simulink model "Full_Integration_Redundant"  (R2022b)
settings: Solver=ode15s  StartTime=0.0  StopTime=30  MaxStep=0.01  RelTol=1e-3
undefined symbols (not defined in the file): Bm1, Bm2, Br, Bsc, Btr, Continuous, G, Im1, Im2, Isw, Jtr, Ke, Ke2, Kl, kp, kr, ks, Ksc, Ksr, Kt, Kt2, ktr, Kv1, Kv2, L1, L2, lf, lr, Mr, N, n, n1, R1, R2, rp, Tfrc, Time, to, Vx, waypoints, z
libraries: simulink_extras x13, ctrlSharedLib x2, simulink x2, robotalgslib x1, slpidlib x1
settings Model: Creator=Timothy  LastModifiedBy=Timothy
settings DebuggingCC: SignalInfNanChecking=error

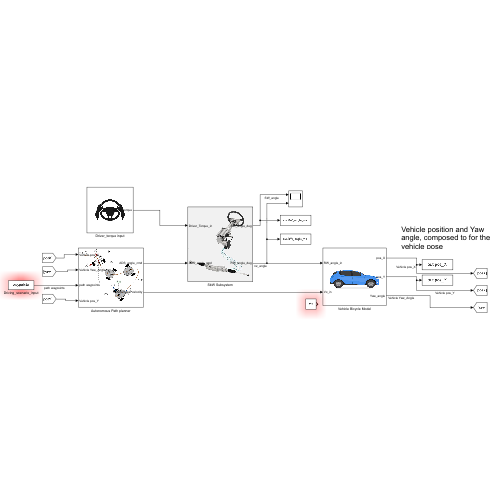
[thumbnail: Simulink's stored preview of the top-level diagram]
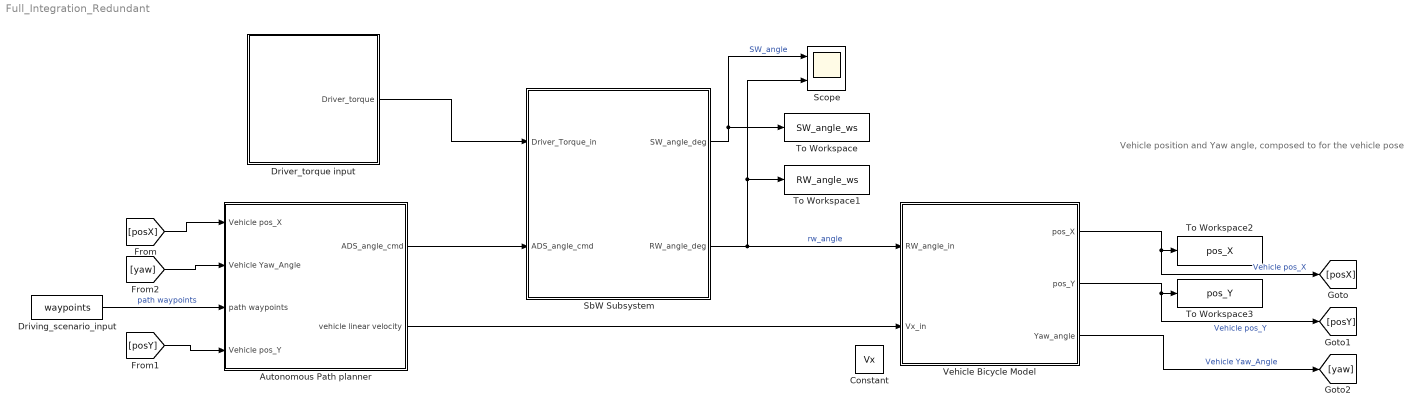
== system Full_Integration_Redundant ==
  note: Vehicle position and Yaw angle, composed to for the vehicle pose
  Autonomous Path planner : Subsystem
      mask Display: image('$imagefile'); % Use "Edit Image" on toolstrip to change.
  Constant : Constant  Value=Vx
  Driver_torque input : Subsystem
      mask Display: image('$imagefile'); % Use "Edit Image" on toolstrip to change.
  Driving_scenario_input : Constant  Value=waypoints
  SbW Subsystem : Subsystem
      mask Display: image('$imagefile'); % Use "Edit Image" on toolstrip to change.
  Scope : Scope  NumInputPorts=2
  To Workspace : ToWorkspace  VariableName=SW_angle_ws  SaveFormat=Timeseries  SampleTime=-1
  To Workspace1 : ToWorkspace  VariableName=RW_angle_ws  SaveFormat=Timeseries  SampleTime=-1
  To Workspace2 : ToWorkspace  VariableName=pos_X  SaveFormat=Timeseries  SampleTime=-1
  To Workspace3 : ToWorkspace  VariableName=pos_Y  SaveFormat=Timeseries  SampleTime=-1
  Vehicle Bicycle Model : Subsystem
      mask Display: image('$imagefile'); % Use "Edit Image" on toolstrip to change.
  wires:
  SbW Subsystem/1(SW_angle_deg) -> Scope/1, To Workspace/1  "SW_angle"
  Driving_scenario_input/1 -> Autonomous Path planner/3(path waypoints)  "path waypoints"
  Vehicle Bicycle Model/2(pos_Y) -> To Workspace3/1, [posY]  "Vehicle pos_Y"
  Autonomous Path planner/1(ADS_angle_cmd) -> SbW Subsystem/2(ADS_angle_cmd)
  Vehicle Bicycle Model/3(Yaw_angle) -> [yaw]  "Vehicle Yaw_Angle"
  SbW Subsystem/2(RW_angle_deg) -> Scope/2, To Workspace1/1, Vehicle Bicycle Model/1(RW_angle_in)  "rw_angle"
  Vehicle Bicycle Model/1(pos_X) -> [posX], To Workspace2/1  "Vehicle pos_X"
  [posX] -> Autonomous Path planner/1(Vehicle pos_X)
  [posY] -> Autonomous Path planner/4(Vehicle pos_Y)
  [yaw] -> Autonomous Path planner/2(Vehicle Yaw_Angle)
  Autonomous Path planner/2(vehicle linear velocity) -> Vehicle Bicycle Model/2(Vx_in)
  Driver_torque input/1(Driver_torque) -> SbW Subsystem/1(Driver_Torque_in)

== system Full_Integration_Redundant/Autonomous Path planner ==
  Vehicle pos_X : Inport
  Vehicle Yaw_Angle : Inport  Port=2
  path waypoints : Inport  Port=3
  Vehicle pos_Y : Inport  Port=4
  Angular converter : MATLAB Function  TreatAsAtomicUnit=on
  Mux : Mux  Inputs=3
  Pure Pursuit : robotalgslib/Pure Pursuit  DesiredLinearVelocity=1.7  MaxAngularVelocity=50  LookaheadDistance=1.0  TargetDirPort=off  SimulateUsing=Code generation
      settings: LibrarySourceBlock=robotmobilelib/Pure Pursuit
  Radians to Degrees : simulink_extras/Transformations/Radians to Degrees
  Scope3 : Scope
  ADS_angle_cmd : Outport
  vehicle linear velocity : Outport  Port=2
  wires:
  Vehicle pos_Y/1 -> Mux/2
  Pure Pursuit/1 -> vehicle linear velocity/1, Scope3/1, Angular converter/2(v)  "vehicle linear velocity"
  Vehicle Yaw_Angle/1 -> Mux/3
  Pure Pursuit/2 -> Angular converter/1(omega)
  Mux/1 -> Pure Pursuit/1  "vehicle_pose"
  Angular converter/1(delta) -> Radians to Degrees/1
  Radians to Degrees/1 -> ADS_angle_cmd/1  "ADS_angle_cmd"
  path waypoints/1 -> Pure Pursuit/2
  Vehicle pos_X/1 -> Mux/1

== system Full_Integration_Redundant/Driver_torque input ==
  note: The Driver torque configuration Can be entered here
  Add : Sum  Inputs=+-+-
  Step : Step  Time=0  SampleTime=0
  Step1 : Step  Time=0  After=0  SampleTime=0
  Step2 : Step  Time=0  After=0  SampleTime=0
  Step3 : Step  Time=0  After=0  SampleTime=0
  Driver_torque : Outport
  wires:
  Step/1 -> Add/1
  Add/1 -> Driver_torque/1  "Driver_torque"
  Step1/1 -> Add/2
  Step2/1 -> Add/3
  Step3/1 -> Add/4

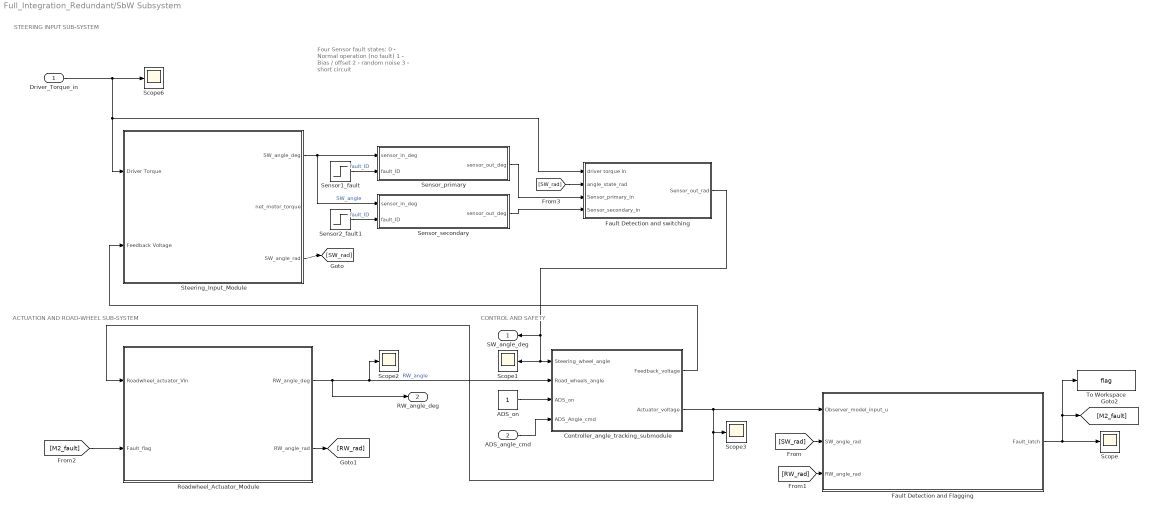
== system Full_Integration_Redundant/SbW Subsystem ==
  note: CONTROL AND SAFETY
  note: Four Sensor fault states:
      | 0 - Normal operation (no fault)
      | 1 - Bias / offset
      | 2 - random noise
      | 3 - short circuit
  note: ACTUATION AND ROAD-WHEEL SUB-SYSTEM
  note: STEERING INPUT SUB-SYSTEM
  Driver_Torque_in : Inport
  ADS_angle_cmd : Inport  Port=2
  ADS_on : Constant
  Controller_angle_tracking_submodule : Subsystem
  Fault Detection and Flagging : Subsystem
  Fault Detection and switching : Subsystem
  Roadwheel_Actuator_Module : Subsystem
  Scope{,1..3,6} (5 alike) : Scope
  Sensor1_fault : Step  SampleTime=0
  Sensor2_fault1 : Step  SampleTime=0
  Sensor_primary : Subsystem
  Sensor_secondary : Subsystem
  Steering_Input_Module : Subsystem
  To Workspace : ToWorkspace  VariableName=flag  SaveFormat=Timeseries  SampleTime=-1
  SW_angle_deg : Outport
  RW_angle_deg : Outport  Port=2
  wires:
  Roadwheel_Actuator_Module/1(RW_angle_deg) -> Controller_angle_tracking_submodule/2(Road_wheels_angle), Scope2/1, RW_angle_deg/1  "RW_angle"
  Controller_angle_tracking_submodule/2(Actuator_voltage) -> Fault Detection and Flagging/1(Observer_model_input_u), Roadwheel_Actuator_Module/1(Roadwheel_actuator_Vin), Scope3/1
  Controller_angle_tracking_submodule/1(Feedback_voltage) -> Steering_Input_Module/2(Feedback Voltage)
  Driver_Torque_in/1 -> Fault Detection and switching/1(driver torque in), Steering_Input_Module/1(Driver Torque), Scope6/1
  Steering_Input_Module/3(SW_angle_rad) -> [SW_rad]
  Roadwheel_Actuator_Module/2(RW_angle_rad) -> [RW_rad]
  Fault Detection and Flagging/1(Fault_latch) -> Scope/1, To Workspace/1, [M2_fault]
  ADS_on/1 -> Controller_angle_tracking_submodule/3(ADS_on)
  ADS_angle_cmd/1 -> Controller_angle_tracking_submodule/4(ADS_Angle_cmd)
  [SW_rad] -> Fault Detection and Flagging/2(SW_angle_rad)
  [RW_rad] -> Fault Detection and Flagging/3(RW_angle_rad)
  [M2_fault] -> Roadwheel_Actuator_Module/2(Fault_flag)
  Sensor1_fault/1 -> Sensor_primary/2(fault_ID)  "fault_ID"
  Sensor2_fault1/1 -> Sensor_secondary/2(fault_ID)  "fault_ID"
  [SW_rad] -> Fault Detection and switching/2(angle_state_rad)
  Sensor_primary/1(sensor_out_deg) -> Fault Detection and switching/3(Sensor_primary_in)
  Sensor_secondary/1(sensor_out_deg) -> Fault Detection and switching/4(Sensor_secondary_in)
  Steering_Input_Module/1(SW_angle_deg) -> Sensor_secondary/1(sensor_in_deg), Sensor_primary/1(sensor_in_deg)  "SW_angle"
  Fault Detection and switching/1(Sensor_out_rad) -> SW_angle_deg/1, Scope1/1, Controller_angle_tracking_submodule/1(Steering_wheel_angle)

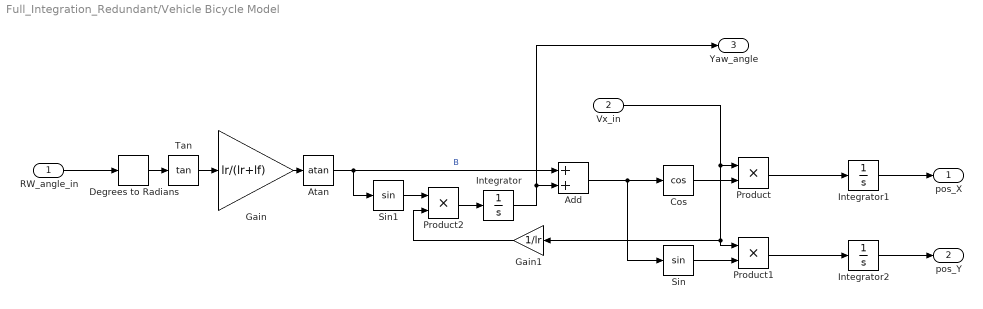
== system Full_Integration_Redundant/Vehicle Bicycle Model ==
  RW_angle_in : Inport
  Vx_in : Inport  Port=2
  Add : Sum
  Atan : Trigonometry  Operator=atan
  Cos : Trigonometry  Operator=cos
  Degrees to Radians : simulink_extras/Transformations/Degrees to Radians
  Gain : Gain  Gain=lr/(lr+lf)
  Gain1 : Gain  Gain=1/lr
  Integrator : Integrator
  Integrator1 : Integrator
  Integrator2 : Integrator
  Product : Product
  Product1 : Product
  Product2 : Product
  Sin : Trigonometry
  Sin1 : Trigonometry
  Tan : Trigonometry  Operator=tan
  pos_X : Outport
  pos_Y : Outport  Port=2
  Yaw_angle : Outport  Port=3
  wires:
  Degrees to Radians/1 -> Tan/1
  Product2/1 -> Integrator/1
  Cos/1 -> Product/2
  Add/1 -> Sin/1, Cos/1
  Atan/1 -> Add/1, Sin1/1  "B"
  Vx_in/1 -> Product1/1, Gain1/1, Product/1
  Integrator1/1 -> pos_X/1
  Gain1/1 -> Product2/2
  Integrator/1 -> Yaw_angle/1, Add/2
  Integrator2/1 -> pos_Y/1
  Gain/1 -> Atan/1
  Product/1 -> Integrator1/1
  Product1/1 -> Integrator2/1
  Tan/1 -> Gain/1
  RW_angle_in/1 -> Degrees to Radians/1
  Sin1/1 -> Product2/1
  Sin/1 -> Product1/2

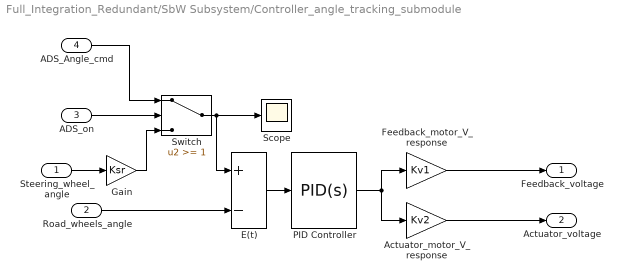
== system Full_Integration_Redundant/SbW Subsystem/Controller_angle_tracking_submodule ==
  Steering_wheel_angle : Inport
  Road_wheels_angle : Inport  Port=2
  ADS_on : Inport  Port=3
  ADS_Angle_cmd : Inport  Port=4
  Actuator_motor_V_response : Gain  Gain=Kv2
  E(t) : Sum  Inputs=+-
  Feedback_motor_V_response : Gain  Gain=Kv1
  Gain : Gain  Gain=Ksr
  PID Controller : slpidlib/PID Controller  Controller=PID  Form=Parallel  TimeDomain=Continuous-time  UseExternalTs=off  SampleTime=-1  IntegratorMethod=Forward Euler  FilterMethod=Forward Euler  ControllerParametersSource=internal  P=27  I=2  UseKiTs=off  D=-0.5  N=100  UseFilter=on  TunerSelectOption=Transfer Function Based (PID Tuner App)  InitialConditionSource=internal  InitialConditionForIntegrator=0  InitialConditionForFilter=0  DifferentiatorICPrevScaledInput=0  ExternalReset=none  TrackingMode=off  Kt=1  LimitOutput=on  SatLimitsSource=internal  UpperSaturationLimit=200  LowerSaturationLimit=-200  LinearizeAsGain=on  AntiWindupMode=back-calculation  Kb=2  LimitIntegrator=on  UpperIntegratorSaturationLimit=inf  LowerIntegratorSaturationLimit=-inf  POutMin=[]  POutMax=[]  IOutMin=[]  IOutMax=[]  DOutMin=[]  DOutMax=[]  NOutMin=[]  NOutMax=[]  SumOutMin=[]  SumOutMax=[]  SaturationOutMin=[]  SaturationOutMax=[]  PParamMin=[]  PParamMax=[]  IParamMin=[]  IParamMax=[]  DParamMin=[]  DParamMax=[]  NParamMin=[]  NParamMax=[]  KbParamMin=[]  KbParamMax=[]  KtParamMin=[]  KtParamMax=[]  KbOutMin=[]  KbOutMax=[]  KtOutMin=[]  KtOutMax=[]  IntegratorOutMin=[]  IntegratorOutMax=[]  FilterOutMin=[]  FilterOutMax=[]  SumI1OutMin=[]  SumI1OutMax=[]  SumI2OutMin=[]  SumI2OutMax=[]  SumI3OutMin=[]  SumI3OutMax=[]  SumI4OutMin=[]  SumI4OutMax=[]  SumDOutMin=[]  SumDOutMax=[]  DifferentiatorOutMin=[]  DifferentiatorOutMax=[]  FilterDiffOutCoefMin=[]  FilterDiffOutCoefMax=[]  ReciprocalOutMin=[]  ReciprocalOutMax=[]  SumDenOutMin=[]  SumDenOutMax=[]  SumNumOutMin=[]  SumNumOutMax=[]  DivideOutMin=[]  DivideOutMax=[]  UdiffTsProdOutMin=[]  UdiffTsProdOutMax=[]  NTsProdOutMin=[]  NTsProdOutMax=[]  UintegralTsProdOutMin=[]  UintegralTsProdOutMax=[]  UngainTsProdOutMin=[]  UngainTsProdOutMax=[]  ClampingZeroOutDataTypeStr=Inherit: Inherit via back propagation  ClampingZeroOutMin=[]  ClampingZeroOutMax=[]  FilterDenConstantOutDataTypeStr=Inherit: Inherit via back propagation  FilterDenConstantOutMin=[]  FilterDenConstantOutMax=[]  PCopyOutDataTypeStr=Inherit: Inherit via back propagation  PCopyOutMin=[]  PCopyOutMax=[]  NCopyOutDataTypeStr=Inherit: Inherit via back propagation  NCopyOutMin=[]  NCopyOutMax=[]  IntegratorContinuousStateAttributes=''  IntegratorStateMustResolveToSignalObject=off  IntegratorRTWStateStorageClass=Auto  FilterContinuousStateAttributes=''  FilterStateMustResolveToSignalObject=off  FilterRTWStateStorageClass=Auto  ParallelPVariant=InternalParameters  IdealPVariant=Disabled  IVariant=InternalParameters  DVariant=InternalParameters  IntegratorVariant=Continuous  SatVariant=Enabled  AWVariant=BackCalculation  PCopyVariant=Disabled  TRVariant=Disabled  FdbkBlocksVariant=Forward  IdealPFdbkVariant=Disabled  SatFdbkVariant=Disabled  DerivativeFilterVariant=ContFilter  NVariant=InternalParameters  NCopyVariant=Disabled  FilterICVariant=InternalICsFilter  IntegratorICVariant=InternalICs  ExternalResetVariant=Disabled  TRSumVariant=Passthrough  SumFdbkVariant=Disabled  SumVariant=Sum_PID  TsampFilterVariant=InternalTs  TsampNgainVariant=Passthrough  TsampIntegralVariant=Passthrough  ExternalSaturationOutDataTypeStr=Inherit: Same as second input
  Scope : Scope
  Switch : Switch  Threshold=1  SaturateOnIntegerOverflow=off  InputSameDT=off
  Feedback_voltage : Outport
  Actuator_voltage : Outport  Port=2
  wires:
  Feedback_motor_V_response/1 -> Feedback_voltage/1
  E(t)/1 -> PID Controller/1
  PID Controller/1 -> Actuator_motor_V_response/1, Feedback_motor_V_response/1
  Road_wheels_angle/1 -> E(t)/2
  Steering_wheel_angle/1 -> Gain/1
  Actuator_motor_V_response/1 -> Actuator_voltage/1
  ADS_on/1 -> Switch/2
  ADS_Angle_cmd/1 -> Switch/1
  Gain/1 -> Switch/3
  Switch/1 -> E(t)/1, Scope/1

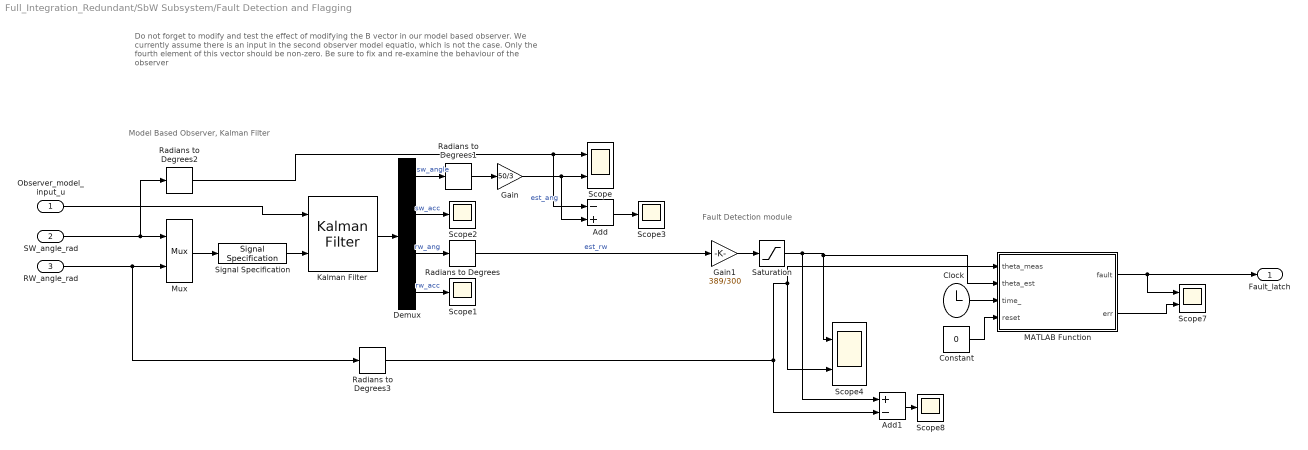
== system Full_Integration_Redundant/SbW Subsystem/Fault Detection and Flagging ==
  note: Do not forget to modify and test the effect of modifying the B vector in our model based observer. We currently assume there is an input in the second observer model equatio, which is not the case. Only the fourth element of this vector should be non-zero. Be sure to fix and re-examine the behaviour of the observer
  note: Fault Detection module
  note: Model Based Observer, Kalman Filter
  Observer_model_input_u : Inport
  SW_angle_rad : Inport  Port=2
  RW_angle_rad : Inport  Port=3
  Add : Sum  Inputs=-+
  Add1 : Sum  Inputs=+-
  Clock : Clock
  Constant : Constant  Value=0
  Demux : Demux
  Gain : Gain  Gain=50/3
  Gain1 : Gain  Gain=389/300
  Kalman Filter : ctrlSharedLib/Kalman Filter  TimeDomain=Continuous-Time  UseCurrentEstimator=on  ModelSource=Individual A, B, C, D matrices  ModelSourceVariable=ss(0.95,1,1,0,1)  A=[0 1 0 0; -(Ksc/Isw) -(Bsc/Isw) (Ksc/Isw) (Bsc/Isw); 0 0 0 1; 0 0 -(Kl/Jtr) -(Btr/Jtr)]  B=[0; 1/Isw; 0; (Kl*z)/(Jtr*N)]  C=[1 0 0 0; 0 0 1 0]  D=0  NumberOfStates=1  NumberOfInputs=1  NumberOfOutputs=1  InitialEstimateSource=Dialog  X0=0  P0=10  UseK=off  UseGH=off  NumberOfProcessNoiseInputs=1  G=1  TimeInvariantG=on  H=0  TimeInvariantH=on  Q=diag([0.01 0.1 0.01 0.1])  TimeInvariantQ=on  R=diag([0.1 0.1])  TimeInvariantR=on  N=0  TimeInvariantN=on  AddInputPort=on  AddEnablePort=off  OutputEstimatedY=off  OutputP=off  Ts=-1
  MATLAB Function : MATLAB Function  TreatAsAtomicUnit=on
  Mux : Mux  Inputs=2
  Radians to Degrees{,1..3} (4 alike) : simulink_extras/Transformations/Radians to Degrees
  Saturation : Saturate  UpperLimit=35  LowerLimit=-35
  Scope : Scope  NumInputPorts=2
  Scope{1..3,8} (4 alike) : Scope
  Scope4 : Scope  NumInputPorts=2
  Scope7 : Scope  NumInputPorts=2
  Signal Specification : SignalSpecification  Dimensions=2
  Fault_latch : Outport
  wires:
  Radians to Degrees3/1 -> Scope4/2, MATLAB Function/1(theta_meas), Add1/2
  Kalman Filter/1 -> Demux/1
  Demux/3 -> Radians to Degrees/1  "rw_ang"
  Demux/1 -> Radians to Degrees1/1  "sw_angle"
  Demux/2 -> Scope2/1  "sw_acc"
  Gain/1 -> Add/2, Scope/2  "est_ang"
  Demux/4 -> Scope1/1  "rw_acc"
  Radians to Degrees/1 -> Gain1/1  "est_rw"
  Mux/1 -> Signal Specification/1
  Add/1 -> Scope3/1
  MATLAB Function/2(err) -> Scope7/2
  Radians to Degrees1/1 -> Gain/1
  Saturation/1 -> Add1/1, MATLAB Function/2(theta_est), Scope4/1
  Constant/1 -> MATLAB Function/4(reset)
  Gain1/1 -> Saturation/1
  Add1/1 -> Scope8/1
  Clock/1 -> MATLAB Function/3(time_)
  MATLAB Function/1(fault) -> Fault_latch/1, Scope7/1
  SW_angle_rad/1 -> Radians to Degrees2/1, Mux/1
  Observer_model_input_u/1 -> Kalman Filter/1
  RW_angle_rad/1 -> Radians to Degrees3/1, Mux/2
  Radians to Degrees2/1 -> Add/1, Scope/1
  Signal Specification/1 -> Kalman Filter/2

== system Full_Integration_Redundant/SbW Subsystem/Fault Detection and switching ==
  driver torque in : Inport
  angle_state_rad : Inport  Port=2
  Sensor_primary_in : Inport  Port=3
  Sensor_secondary_in : Inport  Port=4
  Constant : Constant  Value=0.1
  Kalman Filter : Subsystem
  MATLAB Function : MATLAB Function  TreatAsAtomicUnit=on
  Scope1 : Scope  NumInputPorts=5
  Scope2 : Scope
  Scope3 : Scope
  Sensor_out_rad : Outport
  wires:
  MATLAB Function/2(fault_flag) -> Scope1/2  "Fault_Flag"
  MATLAB Function/3(selected_sensor_id) -> Scope1/3  "Sensor_ID"
  Sensor_primary_in/1 -> Scope1/4, MATLAB Function/1(sensor1), Scope2/1  "Sensor_primary_in"
  Kalman Filter/1(s1) -> MATLAB Function/3(estimated_value)
  MATLAB Function/1(selected_sensor) -> Sensor_out_rad/1, Scope1/1  "Sensor_Output"
  Sensor_secondary_in/1 -> Scope1/5, Scope3/1, MATLAB Function/2(sensor2)
  Constant/1 -> MATLAB Function/4(noise_threshold)
  driver torque in/1 -> Kalman Filter/1(u)
  angle_state_rad/1 -> Kalman Filter/2(y)

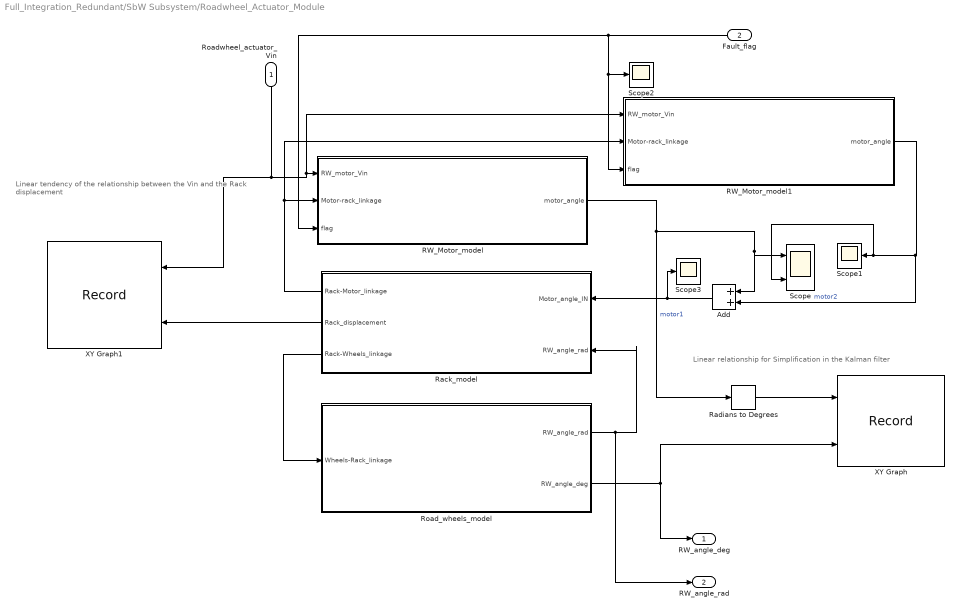
== system Full_Integration_Redundant/SbW Subsystem/Roadwheel_Actuator_Module ==
  note: Linear tendency of the relationship between the
      | Vin and the Rack displacement
  note: Linear relationship for Simplification in the Kalman filter
  Roadwheel_actuator_Vin : Inport
  Fault_flag : Inport  Port=2
  Add : Sum
  RW_Motor_model : Subsystem
  RW_Motor_model1 : Subsystem
  Rack_model : Subsystem
  Radians to Degrees : simulink_extras/Transformations/Radians to Degrees
  Road_wheels_model : Subsystem
  Scope : Scope  NumInputPorts=2
  Scope1 : Scope
  Scope2 : Scope
  Scope3 : Scope
  XY Graph : Record  FileSettingsInternal="{\"entries\":[{\"content\":{\"excelSettings\":{\"content\":{},\"type\":\"Streamout.ExcelSettings\"}},\"type\":\"Streamout.FileSettingStorage\",\"uuid\":\"639db076-b845-40fa-afa2-89a37e17982f\"}],\"packageUris\":[\"http://schema.mathworks.com/mf0/streamout_blocks/R2020a\"],\"version\":\"1.0\"}"  Layout=[1 1]  SignalsInternal="{\"entries\":[{\"content\":{\"signals\":[{\"content\":{\"blockPath\":[\"Full_Integration_Redundant/SbW Subsystem/Roadwheel_Actuator_Module/XY Graph\"],\"channel\":[],\"dimensions\":[1],\"domain\":\"Full_Integration_Redundant/SbW Subsystem/Roadwheel_Actuator_Module/XY Graph\",\"lineColor\":\"#a2142f\",\"plots\":[1],\"port\":1,\"sid\":[],\"signalID\":16,\"signalName\":\"Radians\\nto Degrees\"},\"type\":\"RecordBlkView.Signal\",\"uuid\":\"466d8f2a-f097-4c4d-8963-3db64aae8002\"},{\"content\":{\"blockPath\":[\"Full_Integration_Redundant/SbW Subsystem/Roadwheel_Actuator_Module/XY Graph\"],\"channel\":[],\"dimensions\":[1],\"domain\":\"Full_Integration_Redundant/SbW Subsystem/Roadwheel_Actuator_Module/XY Graph\",\"lineColor\":\"#139fff\",\"plots\":[1],\"port\":2,\"sid\":[],\"signalID\":19,\"signalName\":\"Road_wheels_model:2\"},\"type\":\"RecordBlkView.Signal\",\"uuid\":\"50170aae-890a-412b-97e5-a37d70f2dd25\"}]},\"type\":\"RecordBlkView.InputSignals\",\"uuid\":\"cd6dec31-1972-4dac-bd49-0ac79019fc64\"}],\"packageUris\":[\"http://schema.mathworks.com/mf0/streamout_blocks/R2020a\"],\"version\":\"1.0\"}"  VisualizationBindings="{\"xyplotplugin\":{\"info\":[{\"series\":[{\"bindingParametersList\":[{\"parameter\":\"X-Axis\",\"signalID\":16,\"signalName\":\"Radians\\nto Degrees\"},{\"parameter\":\"Y-Axis\",\"signalID\":19,\"signalName\":\"Road_wheels_model:2\"}],\"seriesID\":30989}],\"subplotID\":1}]}}"  CompatibilityTag=XY
  XY Graph1 : Record  FileSettingsInternal="{\"entries\":[{\"content\":{\"excelSettings\":{\"content\":{},\"type\":\"Streamout.ExcelSettings\"}},\"type\":\"Streamout.FileSettingStorage\",\"uuid\":\"46917eaa-2583-42c8-a8bf-cf8cc34bcc49\"}],\"packageUris\":[\"http://schema.mathworks.com/mf0/streamout_blocks/R2020a\"],\"version\":\"1.0\"}"  Layout=[1 1]  SignalsInternal="{\"entries\":[{\"content\":{\"signals\":[{\"content\":{\"blockPath\":[\"Full_Integration_Redundant/SbW Subsystem/Roadwheel_Actuator_Module/XY Graph1\"],\"channel\":[],\"dimensions\":[1],\"domain\":\"Full_Integration_Redundant/SbW Subsystem/Roadwheel_Actuator_Module/XY Graph1\",\"lineColor\":\"#a2142f\",\"plots\":[1],\"port\":1,\"sid\":[],\"signalID\":8,\"signalName\":\"Roadwheel_actuator_Vin\"},\"type\":\"RecordBlkView.Signal\",\"uuid\":\"14664490-ed74-4463-938d-4ad4b4babf31\"},{\"content\":{\"blockPath\":[\"Full_Integration_Redundant/SbW Subsystem/Roadwheel_Actuator_Module/XY Graph1\"],\"channel\":[],\"dimensions\":[1],\"domain\":\"Full_Integration_Redundant/SbW Subsystem/Roadwheel_Actuator_Module/XY Graph1\",\"lineColor\":\"#139fff\",\"plots\":[1],\"port\":2,\"sid\":[],\"signalID\":11,\"signalName\":\"Rack_model:2\"},\"type\":\"RecordBlkView.Signal\",\"uuid\":\"2dcc45c1-6713-4163-a73d-48023264d737\"}]},\"type\":\"RecordBlkView.InputSignals\",\"uuid\":\"93d8719a-0e2e-4ca8-9771-3c7b9e441b86\"}],\"packageUris\":[\"http://schema.mathworks.com/mf0/streamout_blocks/R2020a\"],\"version\":\"1.0\"}"  VisualizationBindings="{\"xyplotplugin\":{\"info\":[{\"series\":[{\"bindingParametersList\":[{\"parameter\":\"X-Axis\",\"signalID\":8,\"signalName\":\"Roadwheel_actuator_Vin\"},{\"parameter\":\"Y-Axis\",\"signalID\":11,\"signalName\":\"Rack_model:2\"}],\"seriesID\":50607}],\"subplotID\":1}]}}"  CompatibilityTag=XY
  RW_angle_deg : Outport
  RW_angle_rad : Outport  Port=2
  wires:
  Roadwheel_actuator_Vin/1 -> RW_Motor_model1/1(RW_motor_Vin), RW_Motor_model/1(RW_motor_Vin), XY Graph1/1
  Rack_model/1(Rack-Motor_linkage) -> RW_Motor_model1/2(Motor-rack_linkage), RW_Motor_model/2(Motor-rack_linkage)
  Rack_model/3(Rack-Wheels_linkage) -> Road_wheels_model/1(Wheels-Rack_linkage)
  Road_wheels_model/1(RW_angle_rad) -> RW_angle_rad/1, Rack_model/2(RW_angle_rad)
  Road_wheels_model/2(RW_angle_deg) -> XY Graph/2, RW_angle_deg/1
  RW_Motor_model/1(motor_angle) -> Radians to Degrees/1, Add/1, Scope/1  "motor1"
  Radians to Degrees/1 -> XY Graph/1
  Rack_model/2(Rack_displacement) -> XY Graph1/2
  Fault_flag/1 -> RW_Motor_model/3(flag), Scope2/1, RW_Motor_model1/3(flag)
  RW_Motor_model1/1(motor_angle) -> Add/2, Scope/2, Scope1/1  "motor2"
  Add/1 -> Scope3/1, Rack_model/1(Motor_angle_IN)

== system Full_Integration_Redundant/SbW Subsystem/Sensor_primary ==
  sensor_in_deg : Inport
  fault_ID : Inport  Port=2
  Degrees to Radians : simulink_extras/Transformations/Degrees to Radians
  MATLAB Function2 : MATLAB Function  TreatAsAtomicUnit=on
  Radians to Degrees : simulink_extras/Transformations/Radians to Degrees
  Sensor : Subsystem
  sensor_out_deg : Outport
  wires:
  Sensor/1(actaul_angle_degre) -> MATLAB Function2/1(sensor_in)
  MATLAB Function2/1(sensor_out) -> Radians to Degrees/1  "sensor_out_rad"
  sensor_in_deg/1 -> Degrees to Radians/1
  fault_ID/1 -> MATLAB Function2/2(fault_type)
  Degrees to Radians/1 -> Sensor/1(SW_angle_rad)
  Radians to Degrees/1 -> sensor_out_deg/1

== system Full_Integration_Redundant/SbW Subsystem/Sensor_secondary ==
  sensor_in_deg : Inport
  fault_ID : Inport  Port=2
  Degrees to Radians : simulink_extras/Transformations/Degrees to Radians
  MATLAB Function2 : MATLAB Function  TreatAsAtomicUnit=on
  Radians to Degrees : simulink_extras/Transformations/Radians to Degrees
  Sensor : Subsystem
  sensor_out_deg : Outport
  wires:
  Radians to Degrees/1 -> sensor_out_deg/1
  Degrees to Radians/1 -> Sensor/1(SW_angle_rad)
  fault_ID/1 -> MATLAB Function2/2(fault_type)
  sensor_in_deg/1 -> Degrees to Radians/1
  MATLAB Function2/1(sensor_out) -> Radians to Degrees/1  "sensor_out_rad"
  Sensor/1(actaul_angle_degre) -> MATLAB Function2/1(sensor_in)

== system Full_Integration_Redundant/SbW Subsystem/Steering_Input_Module ==
  Driver Torque : Inport
  Feedback Voltage : Inport  Port=2
  SW_Motor_model : Subsystem
  Scope : Scope
  Steering_wheel_model : Subsystem
  net_torque : Sum
  SW_angle_deg : Outport
  net_motor_torque : Outport  Port=2
  SW_angle_rad : Outport  Port=3
  wires:
  Driver Torque/1 -> net_torque/1, Steering_wheel_model/1(Torque_in)
  Steering_wheel_model/1(SW_angle_deg) -> SW_angle_deg/1
  Steering_wheel_model/2(SW_ang_vel) -> SW_Motor_model/1(SW_ang_vel)
  Steering_wheel_model/3(SW_angle_rad) -> SW_angle_rad/1, SW_Motor_model/2(SW_angle_rad)
  Feedback Voltage/1 -> SW_Motor_model/3(SW_motor_Vin)
  SW_Motor_model/1(Motor_ang_vel) -> Steering_wheel_model/2(SW_motor_angular_velocity)
  SW_Motor_model/2(Motor_pos) -> Steering_wheel_model/3(SW_motor_position)
  SW_Motor_model/3(feedback_torque) -> net_torque/2
  net_torque/1 -> Scope/1, net_motor_torque/1

== system Full_Integration_Redundant/SbW Subsystem/Fault Detection and switching/Kalman Filter ==
  u : Inport
  y : Inport  Port=2
  Demux : Demux
  Kalman Filter1 : ctrlSharedLib/Kalman Filter  TimeDomain=Continuous-Time  UseCurrentEstimator=on  ModelSource=Individual A, B, C, D matrices  ModelSourceVariable=sys  A=[0 1 0 0; -(Ksc/Isw) -(Bsc/Isw) (Ksc/Isw) (Bsc/Isw); 0 0 0 1; (Ksc/Im1) (Bsc/Im1) -(Ksc/Im1) -(Bsc+Bm1)/(Im1)]  B=[0; 1/Isw; 0; 1/Im1]  C=[1 0 0 0]  D=0  NumberOfStates=2  NumberOfInputs=2  NumberOfOutputs=2  InitialEstimateSource=Dialog  X0=0  P0=10  UseK=off  UseGH=off  NumberOfProcessNoiseInputs=2  G=1  TimeInvariantG=on  H=0  TimeInvariantH=on  Q="diag([1e-6   1e-4   1e-6   1e-3])"  TimeInvariantQ=on  R=0.0001  TimeInvariantR=on  N=0  TimeInvariantN=on  AddInputPort=on  AddEnablePort=off  OutputEstimatedY=off  OutputP=off  Ts=-1
  Saturation : Saturate  UpperLimit=7.85  LowerLimit=-7.85
  Scope{1,6..8} (4 alike) : Scope
  s1 : Outport
  wires:
  Kalman Filter1/1 -> Demux/1  "estimate_angle"
  Demux/1 -> Scope1/1, Saturation/1
  Demux/2 -> Scope6/1
  y/1 -> Kalman Filter1/2
  u/1 -> Kalman Filter1/1
  Saturation/1 -> s1/1
  Demux/3 -> Scope7/1
  Demux/4 -> Scope8/1

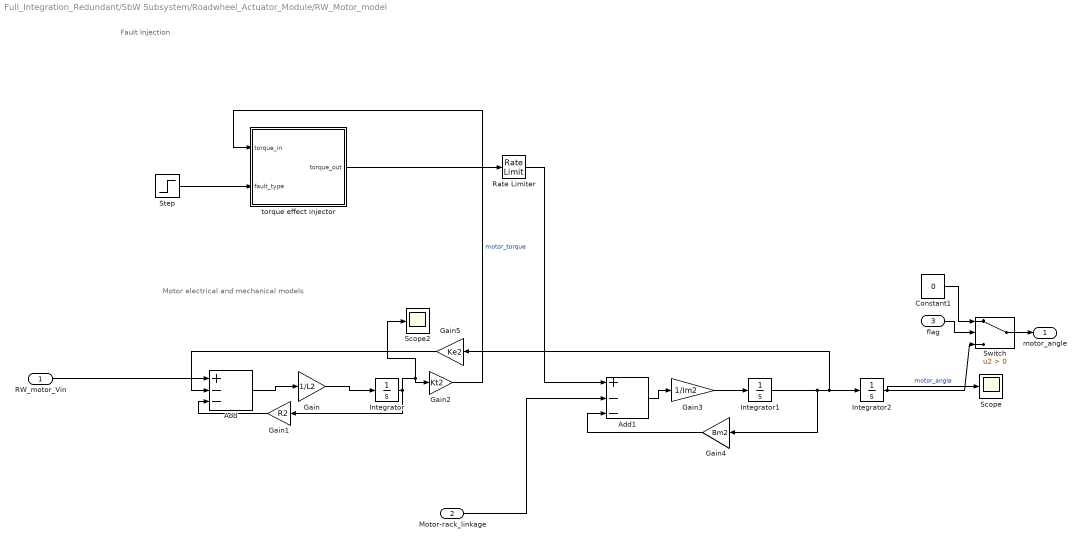
== system Full_Integration_Redundant/SbW Subsystem/Roadwheel_Actuator_Module/RW_Motor_model ==
  note: Fault Injection
  note: Motor electrical and mechanical models
  RW_motor_Vin : Inport
  Motor-rack_linkage : Inport  Port=2
  flag : Inport  Port=3
  Add : Sum  Inputs=+--
  Add1 : Sum  Inputs=+--
  Constant1 : Constant  Value=0
  Gain : Gain  Gain=1/L2
  Gain1 : Gain  Gain=R2
  Gain2 : Gain  Gain=Kt2
  Gain3 : Gain  Gain=1/Im2
  Gain4 : Gain  Gain=Bm2
  Gain5 : Gain  Gain=Ke2
  Integrator : Integrator
  Integrator1 : Integrator
  Integrator2 : Integrator
  Rate Limiter : RateLimiter  RisingSlewLimit=20  FallingSlewLimit=-20  SampleTimeMode=inherited
  Scope : Scope
  Scope2 : Scope
  Step : Step  Time=10  After=0  SampleTime=0
  Switch : Switch  Criteria=u2 > Threshold  SaturateOnIntegerOverflow=off  InputSameDT=off
  torque effect injector : MATLAB Function  TreatAsAtomicUnit=on
  motor_angle : Outport
  wires:
  Gain3/1 -> Integrator1/1
  Gain4/1 -> Add1/3
  Integrator1/1 -> Gain4/1, Gain5/1, Integrator2/1
  Integrator2/1 -> Scope/1, Switch/3  "motor_angle"
  Gain/1 -> Integrator/1
  Integrator/1 -> Gain1/1, Gain2/1, Scope2/1
  Add1/1 -> Gain3/1
  Gain5/1 -> Add/2
  Gain1/1 -> Add/3
  Add/1 -> Gain/1
  Motor-rack_linkage/1 -> Add1/2
  RW_motor_Vin/1 -> Add/1
  Gain2/1 -> torque effect injector/1(torque_in)  "motor_torque"
  torque effect injector/1(torque_out) -> Rate Limiter/1
  flag/1 -> Switch/2
  Constant1/1 -> Switch/1
  Switch/1 -> motor_angle/1
  Step/1 -> torque effect injector/2(fault_type)
  Rate Limiter/1 -> Add1/1

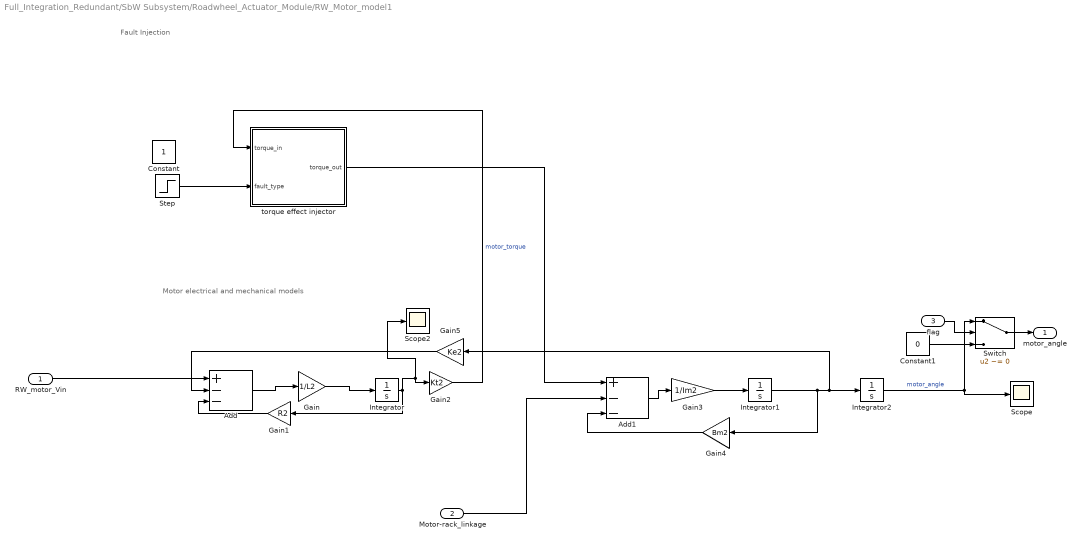
== system Full_Integration_Redundant/SbW Subsystem/Roadwheel_Actuator_Module/RW_Motor_model1 ==
  note: Fault Injection
  note: Motor electrical and mechanical models
  RW_motor_Vin : Inport
  Motor-rack_linkage : Inport  Port=2
  flag : Inport  Port=3
  Add : Sum  Inputs=+--
  Add1 : Sum  Inputs=+--
  Constant : Constant
  Constant1 : Constant  Value=0
  Gain : Gain  Gain=1/L2
  Gain1 : Gain  Gain=R2
  Gain2 : Gain  Gain=Kt2
  Gain3 : Gain  Gain=1/Im2
  Gain4 : Gain  Gain=Bm2
  Gain5 : Gain  Gain=Ke2
  Integrator : Integrator
  Integrator1 : Integrator
  Integrator2 : Integrator
  Scope : Scope
  Scope2 : Scope
  Step : Step  Time=10  After=0  SampleTime=0
  Switch : Switch  Criteria=u2 ~= 0  SaturateOnIntegerOverflow=off  InputSameDT=off
  torque effect injector : MATLAB Function  TreatAsAtomicUnit=on
  motor_angle : Outport
  wires:
  Gain3/1 -> Integrator1/1
  Gain4/1 -> Add1/3
  Gain/1 -> Integrator/1
  Integrator/1 -> Gain1/1, Gain2/1, Scope2/1
  Add1/1 -> Gain3/1
  Gain5/1 -> Add/2
  Gain1/1 -> Add/3
  Add/1 -> Gain/1
  Motor-rack_linkage/1 -> Add1/2
  RW_motor_Vin/1 -> Add/1
  Gain2/1 -> torque effect injector/1(torque_in)  "motor_torque"
  torque effect injector/1(torque_out) -> Add1/1
  flag/1 -> Switch/2
  Switch/1 -> motor_angle/1
  Step/1 -> torque effect injector/2(fault_type)
  Integrator2/1 -> Scope/1, Switch/1  "motor_angle"
  Constant1/1 -> Switch/3
  Integrator1/1 -> Gain4/1, Gain5/1, Integrator2/1

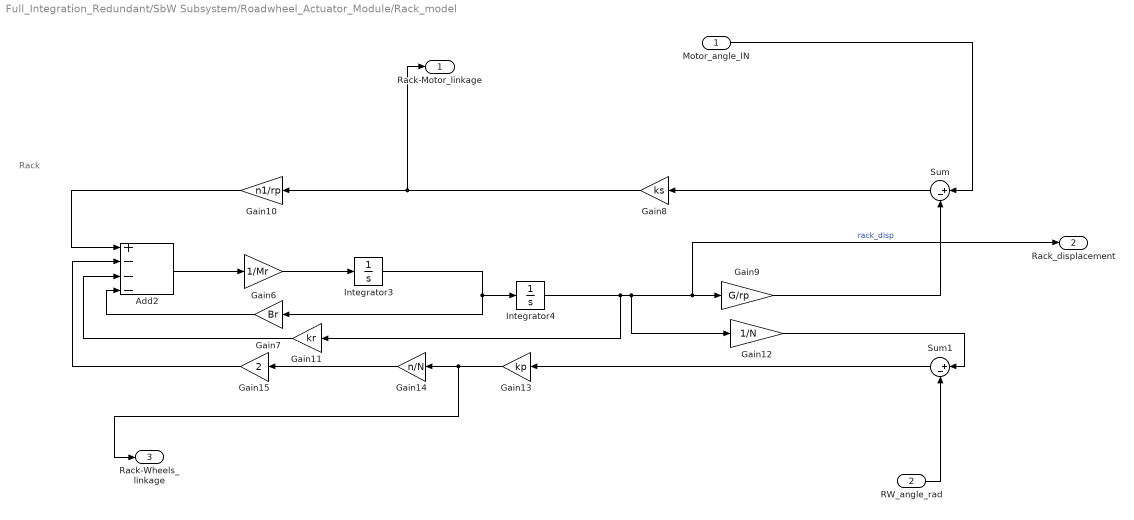
== system Full_Integration_Redundant/SbW Subsystem/Roadwheel_Actuator_Module/Rack_model ==
  note: Rack
  Motor_angle_IN : Inport
  RW_angle_rad : Inport  Port=2
  Add2 : Sum  Inputs=+---
  Gain10 : Gain  Gain=n1/rp
  Gain11 : Gain  Gain=kr
  Gain12 : Gain  Gain=1/N
  Gain13 : Gain  Gain=kp
  Gain14 : Gain  Gain=n/N
  Gain15 : Gain  Gain=2
  Gain6 : Gain  Gain=1/Mr
  Gain7 : Gain  Gain=Br
  Gain8 : Gain  Gain=ks
  Gain9 : Gain  Gain=G/rp
  Integrator3 : Integrator
  Integrator4 : Integrator
  Sum : Sum  Inputs=|+-
  Sum1 : Sum  Inputs=|+-
  Rack-Motor_linkage : Outport
  Rack_displacement : Outport  Port=2
  Rack-Wheels_linkage : Outport  Port=3
  wires:
  RW_angle_rad/1 -> Sum1/2
  Gain10/1 -> Add2/1
  Gain8/1 -> Rack-Motor_linkage/1, Gain10/1
  Integrator4/1 -> Gain11/1, Gain12/1, Rack_displacement/1, Gain9/1  "rack_disp"
  Sum1/1 -> Gain13/1
  Gain9/1 -> Sum/2
  Add2/1 -> Gain6/1
  Integrator3/1 -> Gain7/1, Integrator4/1
  Gain7/1 -> Add2/4
  Gain12/1 -> Sum1/1
  Gain14/1 -> Gain15/1
  Sum/1 -> Gain8/1
  Motor_angle_IN/1 -> Sum/1
  Gain11/1 -> Add2/3
  Gain13/1 -> Rack-Wheels_linkage/1, Gain14/1
  Gain6/1 -> Integrator3/1
  Gain15/1 -> Add2/2

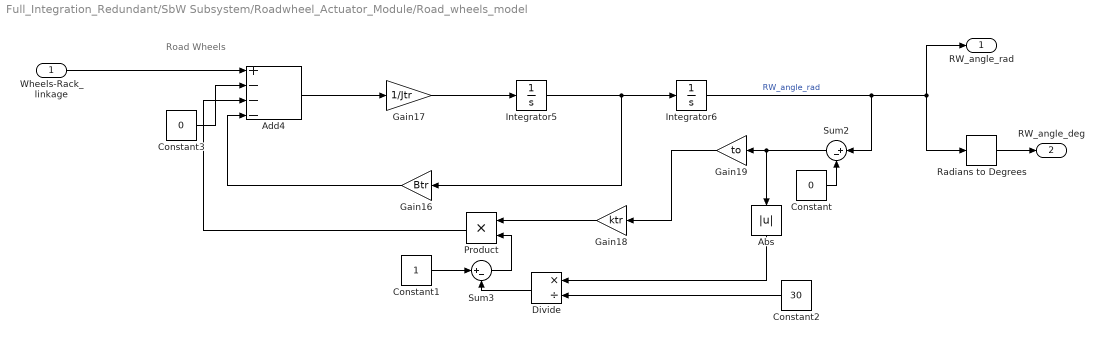
== system Full_Integration_Redundant/SbW Subsystem/Roadwheel_Actuator_Module/Road_wheels_model ==
  note: Road Wheels
  Wheels-Rack_linkage : Inport
  Abs : Abs  SaturateOnIntegerOverflow=off
  Add4 : Sum  Inputs=+---
  Constant : Constant  Value=0
  Constant1 : Constant
  Constant2 : Constant  Value=30
  Constant3 : Constant  Value=0
  Divide : Product  Inputs=*/
  Gain16 : Gain  Gain=Btr
  Gain17 : Gain  Gain=1/Jtr
  Gain18 : Gain  Gain=ktr
  Gain19 : Gain  Gain=to
  Integrator5 : Integrator
  Integrator6 : Integrator
  Product : Product
  Radians to Degrees : simulink_extras/Transformations/Radians to Degrees
  Sum2 : Sum  Inputs=|+-
  Sum3 : Sum  Inputs=|+-
  RW_angle_rad : Outport
  RW_angle_deg : Outport  Port=2
  wires:
  Integrator5/1 -> Gain16/1, Integrator6/1
  Constant/1 -> Sum2/2
  Abs/1 -> Divide/1
  Sum3/1 -> Product/2
  Constant1/1 -> Sum3/1
  Gain18/1 -> Product/1
  Divide/1 -> Sum3/2
  Gain16/1 -> Add4/4
  Gain17/1 -> Integrator5/1
  Constant3/1 -> Add4/2
  Gain19/1 -> Gain18/1
  Constant2/1 -> Divide/2
  Product/1 -> Add4/3
  Sum2/1 -> Abs/1, Gain19/1
  Integrator6/1 -> RW_angle_rad/1, Radians to Degrees/1, Sum2/1  "RW_angle_rad"
  Wheels-Rack_linkage/1 -> Add4/1
  Add4/1 -> Gain17/1
  Radians to Degrees/1 -> RW_angle_deg/1

== system Full_Integration_Redundant/SbW Subsystem/Sensor_primary/Sensor ==
  SW_angle_rad : Inport
  Band-Limited White Noise : simulink/Sources/Band-Limited White Noise  Cov=0  Ts=0.01  seed=[23341]
  Constant : Constant  Value=0.00000001  SampleTime=0.01
  Gain : Gain
  Saturation : Saturate  UpperLimit=7.85  LowerLimit=-7.85
  Sum : Sum  Inputs=|++
  Sum1 : Sum  Inputs=|++
  actaul_angle_degre : Outport
  wires:
  Gain/1 -> Sum/1
  Sum/1 -> Sum1/1
  Constant/1 -> Sum/2
  Sum1/1 -> Saturation/1  "actaul_angle_degre"
  SW_angle_rad/1 -> Gain/1
  Band-Limited White Noise/1 -> Sum1/2
  Saturation/1 -> actaul_angle_degre/1

== system Full_Integration_Redundant/SbW Subsystem/Sensor_secondary/Sensor ==
  SW_angle_rad : Inport
  Band-Limited White Noise : simulink/Sources/Band-Limited White Noise  Cov=0  Ts=0.01  seed=[23341]
  Constant : Constant  Value=0.00000001  SampleTime=0.01
  Gain : Gain
  Saturation : Saturate  UpperLimit=7.85  LowerLimit=-7.85
  Sum : Sum  Inputs=|++
  Sum1 : Sum  Inputs=|++
  actaul_angle_degre : Outport
  wires:
  Saturation/1 -> actaul_angle_degre/1
  Band-Limited White Noise/1 -> Sum1/2
  SW_angle_rad/1 -> Gain/1
  Sum1/1 -> Saturation/1  "actaul_angle_degre"
  Constant/1 -> Sum/2
  Sum/1 -> Sum1/1
  Gain/1 -> Sum/1

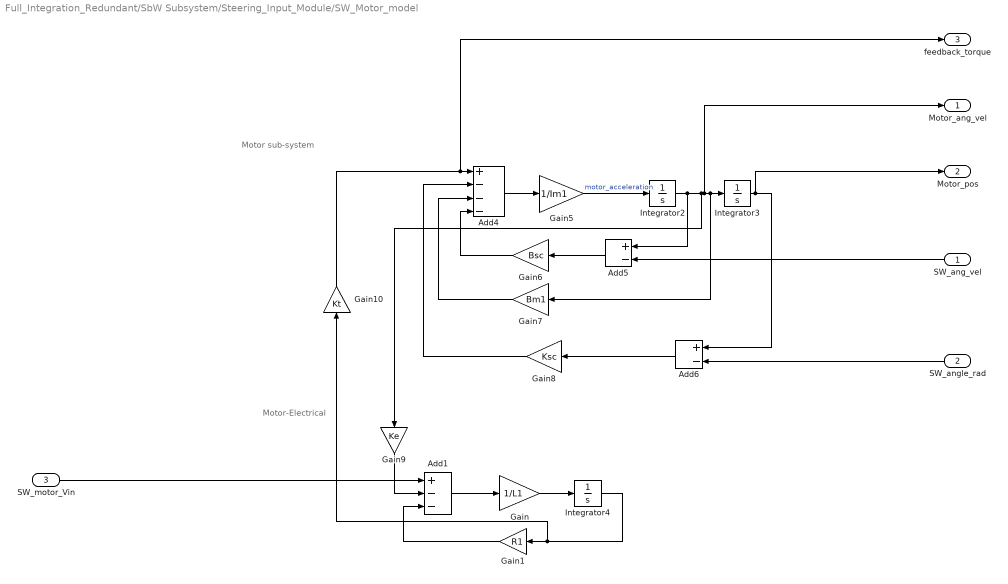
== system Full_Integration_Redundant/SbW Subsystem/Steering_Input_Module/SW_Motor_model ==
  note: Motor-Electrical
  note: Motor sub-system
  SW_ang_vel : Inport
  SW_angle_rad : Inport  Port=2
  SW_motor_Vin : Inport  Port=3
  Add1 : Sum  Inputs=+--
  Add4 : Sum  Inputs=+---
  Add5 : Sum  Inputs=+-
  Add6 : Sum  Inputs=+-
  Gain : Gain  Gain=1/L1
  Gain1 : Gain  Gain=R1
  Gain10 : Gain  Gain=Kt
  Gain5 : Gain  Gain=1/Im1
  Gain6 : Gain  Gain=Bsc
  Gain7 : Gain  Gain=Bm1
  Gain8 : Gain  Gain=Ksc
  Gain9 : Gain  Gain=Ke
  Integrator2 : Integrator
  Integrator3 : Integrator
  Integrator4 : Integrator
  Motor_ang_vel : Outport
  Motor_pos : Outport  Port=2
  feedback_torque : Outport  Port=3
  wires:
  Gain7/1 -> Add4/3
  Gain10/1 -> feedback_torque/1, Add4/1
  Gain8/1 -> Add4/2
  Add5/1 -> Gain6/1
  Integrator2/1 -> Gain9/1, Motor_ang_vel/1, Gain7/1, Integrator3/1, Add5/1
  Gain9/1 -> Add1/2
  Gain5/1 -> Integrator2/1  "motor_acceleration"
  Gain6/1 -> Add4/4
  SW_ang_vel/1 -> Add5/2
  SW_motor_Vin/1 -> Add1/1
  Integrator4/1 -> Gain1/1, Gain10/1
  Gain/1 -> Integrator4/1
  Add6/1 -> Gain8/1
  Integrator3/1 -> Motor_pos/1, Add6/1
  Add1/1 -> Gain/1
  Gain1/1 -> Add1/3
  Add4/1 -> Gain5/1
  SW_angle_rad/1 -> Add6/2

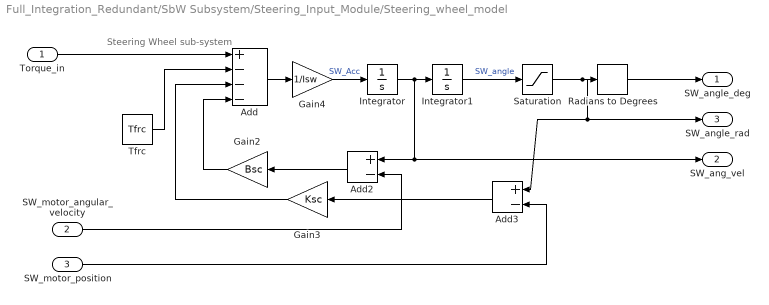
== system Full_Integration_Redundant/SbW Subsystem/Steering_Input_Module/Steering_wheel_model ==
  note: Steering Wheel sub-system
  Torque_in : Inport
  SW_motor_angular_velocity : Inport  Port=2
  SW_motor_position : Inport  Port=3
  Add : Sum  Inputs=+---
  Add2 : Sum  Inputs=+-
  Add3 : Sum  Inputs=+-
  Gain2 : Gain  Gain=Bsc
  Gain3 : Gain  Gain=Ksc
  Gain4 : Gain  Gain=1/Isw
  Integrator : Integrator
  Integrator1 : Integrator
  Radians to Degrees : simulink_extras/Transformations/Radians to Degrees
  Saturation : Saturate  UpperLimit=7.85398  LowerLimit=-7.85398
  Tfrc : Constant  Value=Tfrc
  SW_angle_deg : Outport
  SW_ang_vel : Outport  Port=2
  SW_angle_rad : Outport  Port=3
  wires:
  Tfrc/1 -> Add/2
  Gain4/1 -> Integrator/1  "SW_Acc"
  Integrator1/1 -> Saturation/1  "SW_angle"
  Integrator/1 -> Integrator1/1, SW_ang_vel/1, Add2/1
  Add/1 -> Gain4/1
  Gain2/1 -> Add/4
  Add3/1 -> Gain3/1
  Add2/1 -> Gain2/1
  Gain3/1 -> Add/3
  Radians to Degrees/1 -> SW_angle_deg/1
  SW_motor_angular_velocity/1 -> Add2/2
  SW_motor_position/1 -> Add3/2
  Torque_in/1 -> Add/1
  Saturation/1 -> Add3/1, SW_angle_rad/1, Radians to Degrees/1

== matlab function Full_Integration_Redundant/SbW Subsystem/Fault Detection and Flagging/MATLAB Function ==
  settings: updateMethod=DISCRETE
  data: theta_meas input; fault output; theta_est input; time_ input; reset input; err output
function [fault, err] = fault_detector(theta_meas, theta_est, time_, reset)
%#codegen

% ==============================
% PARAMETERS (tune as needed)
% ==============================
threshold_deg = 7;     % Error threshold in degrees
time_threshold = 0.2;  % Time the error must persist (seconds)

% ==============================
% PERSISTENT VARIABLES
% ==============================
persistent fault_latched;
persistent start_time;
persistent timing_active;

% Initialize persistent variables
if isempty(fault_latched)
    fault_latched = 0;
end

if isempty(start_time)
    start_time = 0;
end

if isempty(timing_active)
    timing_active = 0;
end

% ==============================
% ERROR COMPUTATION
% ==============================
% Convert to degrees no more (assuming inputs are in degrees)
error = abs(theta_est - theta_meas);
err = error;

% ==============================
% RESET LOGIC
% ==============================
if reset == 1
    fault_latched = 0;
    timing_active = 0;
    start_time = 0;
end

% ==============================
% FAULT DETECTION LOGIC
% ==============================
if fault_latched == 0
    
    
    if error > threshold_deg
        
        % Start timing if not already started
        if timing_active == 0
            start_time = time_;
            timing_active = 1;
        end
        
        % Check how long error has persisted
        if (time_ - start_time) >= time_threshold
            fault_latched = 1;
        end
        
    else
        % Error dropped below threshold → reset timing
        timing_active = 0;
        start_time = 0;
    end
    
end

% ==============================
% OUTPUT
% ==============================
fault = fault_latched;

== matlab function Full_Integration_Redundant/SbW Subsystem/Roadwheel_Actuator_Module/RW_Motor_model/torque effect injector ==
  data: torque_in input; torque_out output; fault_type input
% case 0: No fault at all

% case 1: Complete failure, the torque output remains zero
% irrespective of the input

% case 2: weak motor/ reduced torque

function torque_out = motor_fault(torque_in, fault_type)

switch fault_type
    case 0
        torque_out = torque_in; % normal
    case 1
        torque_out = 0; % complete failure
    case 2
        torque_out = 0.7 * torque_in; % weak motor
    otherwise
        torque_out = torque_in;
end

== matlab function Full_Integration_Redundant/SbW Subsystem/Roadwheel_Actuator_Module/RW_Motor_model1/torque effect injector ==
  data: torque_in input; torque_out output; fault_type input
% case 0: No fault at all

% case 1: Complete failure, the torque output remains zero
% irrespective of the input

% case 2: weak motor/ reduced torque

function torque_out = motor_fault(torque_in, fault_type)

switch fault_type
    case 0
        torque_out = torque_in; % normal
    case 1
        torque_out = 0; % complete failure
    case 2
        torque_out = 0.7 * torque_in; % weak motor
    otherwise
        torque_out = torque_in;
end

== matlab function Full_Integration_Redundant/Autonomous Path planner/Angular converter ==
  data: omega input; delta output; v input
function delta = convert(omega, v)

L = 2.5; % <-- set your wheelbase

% Avoid division by zero
if abs(v) < 0.1
    v = 0.1;
end

% delta = atan(L * omega / v);
delta = atan(L * omega / max(v, 0.1));
delta = max(min(delta, 0.9), -0.9);

end

== matlab function Full_Integration_Redundant/SbW Subsystem/Sensor_secondary/MATLAB Function2 ==
  settings: updateMethod=DISCRETE
  data: sensor_in input; sensor_out output; fault_type input


function sensor_out = sensor_fault(sensor_in, fault_type)
% SENSOR_FAULT - Inject sensor faults via Step block
%
% Fault Types:
%   0 = Normal        - clean pass-through
%   1 = Bias          - constant offset added
%   2 = Noise         - random noise added
%   3 = Short Circuit - output forced to zero
%   4 = Drift         - gradual ramp added over time
%
% Connect a Step block to fault_type input:
%   Initial value = 0, Final value = 1/2/3/4

persistent drift_accumulator fault_active stuck_value

% INITIALISATION
if isempty(drift_accumulator)
    drift_accumulator = 0;
    fault_active      = false;
    stuck_value       = 0;
end

% PARAMETERS  – tune these to your signal range
BIAS_VALUE  = 5.0;    % Constant offset for bias fault
NOISE_STD   = 3.0;    % Standard deviation of injected noise
DRIFT_RATE  = 0.05;   % Drift added per sample when fault is active

% Box-Muller noise (replaces randn - works in Simulink Function blocks)
u1 = rand();
u2 = rand();
if u1 < 1e-10; u1 = 1e-10; end
noise = NOISE_STD * sqrt(-2.0 * log(u1)) * cos(2.0 * pi * u2);

% FAULT INJECTION
 
switch round(fault_type)

    case 0
        % NORMAL - clean signal, reset all fault states
        sensor_out        = sensor_in;
        drift_accumulator = 0;
        fault_active      = false;
        stuck_value       = 0;

    case 1
        % BIAS - fixed constant offset
        sensor_out = sensor_in + BIAS_VALUE;

    case 2
        % NOISE - random noise on every sample
        sensor_out = sensor_in + noise;

    case 3
        % SHORT CIRCUIT - output collapses to zero
        sensor_out = 0;

    case 4
        % DRIFT - ramp that grows from the moment Step fires
        if ~fault_active
            fault_active      = true;
            drift_accumulator = 0;   % start ramp from zero at fault onset
        end
        drift_accumulator = drift_accumulator + DRIFT_RATE;
        sensor_out        = sensor_in + drift_accumulator;

    otherwise
        sensor_out = sensor_in;

end
end

== matlab function Full_Integration_Redundant/SbW Subsystem/Fault Detection and switching/MATLAB Function ==
  settings: updateMethod=DISCRETE  sampleTime=0.01
  data: selected_sensor output; sensor1 input; fault_flag output; sensor2 input; estimated_value input; selected_sensor_id output; noise_threshold input
function [selected_sensor, fault_flag, selected_sensor_id] = ...
         sensor_fault_detection(sensor1, sensor2, estimated_value, noise_threshold)

MAX_VAL =  7.85;
MIN_VAL = -7.85;

BUFFER_SIZE           = 30;
FAULT_CONFIRMATION    = 15;
RECOVERY_CONFIRMATION = 50;

INTER_SENSOR_THR = 3.0;
NOISE_THR        = noise_threshold;
SC_ZERO          = 0.3;
SC_MOTION        = 0.5;

persistent buf1 buf2 bufdiff
persistent fc1 fc2
persistent locked1 locked2
persistent sample_count

if isempty(buf1)
    buf1         = ones(BUFFER_SIZE, 1) * sensor1;
    buf2         = ones(BUFFER_SIZE, 1) * sensor2;
    bufdiff      = zeros(BUFFER_SIZE, 1);
    fc1          = 0;     fc2     = 0;
    locked1      = false; locked2 = false;
    sample_count = 0;
end

sample_count = sample_count + 1;

buf1    = [buf1(2:end);    sensor1];
buf2    = [buf2(2:end);    sensor2];
bufdiff = [bufdiff(2:end); abs(sensor1 - sensor2)];

% Suppress until buffer fully populated
if sample_count <= BUFFER_SIZE
    selected_sensor    = clamp(mean(buf1), MIN_VAL, MAX_VAL);
    selected_sensor_id = 1;
    fault_flag         = 0;
    return
end

mn1    = mean(buf1);
mn2    = mean(buf2);
sd1    = std(buf1);
sd2    = std(buf2);
mndiff = mean(bufdiff);

% Fault indicators
s1_noisy = sd1 > NOISE_THR;
s2_noisy = sd2 > NOISE_THR;

s1_short = abs(mn1) < SC_ZERO && abs(mn2) > SC_MOTION;
s2_short = abs(mn2) < SC_ZERO && abs(mn1) > SC_MOTION;

sensors_disagree = mndiff > INTER_SENSOR_THR;
if sensors_disagree
    dist1_from_est = abs(mn1 - estimated_value);
    dist2_from_est = abs(mn2 - estimated_value);
    if dist1_from_est > dist2_from_est
        s1_bias_or_drift = true;
        s2_bias_or_drift = false;
    else
        s1_bias_or_drift = false;
        s2_bias_or_drift = true;
    end
else
    s1_bias_or_drift = false;
    s2_bias_or_drift = false;
end

f1 = s1_noisy || s1_short || s1_bias_or_drift;
f2 = s2_noisy || s2_short || s2_bias_or_drift;

% Lock logic sensor 1 
if ~locked1
    if f1
        fc1 = fc1 + 1;
        if fc1 >= FAULT_CONFIRMATION
            locked1 = true;
            fc1     = 0;
        end
    else
        fc1 = max(fc1 - 1, 0);
    end
else
    if ~f1
        fc1 = fc1 + 1;
        if fc1 >= RECOVERY_CONFIRMATION
            locked1 = false;
            fc1     = 0;
        end
    else
        fc1 = max(fc1 - 1, 0);
    end
end

% Lock logic sensor 2 
if ~locked2
    if f2
        fc2 = fc2 + 1;
        if fc2 >= FAULT_CONFIRMATION
            locked2 = true;
            fc2     = 0;
        end
    else
        fc2 = max(fc2 - 1, 0);
    end
else
    if ~f2
        fc2 = fc2 + 1;
        if fc2 >= RECOVERY_CONFIRMATION
            locked2 = false;
            fc2     = 0;
        end
    else
        fc2 = max(fc2 - 1, 0);
    end
end

% Output selection 
% Locks: permanent exclusion after confirmation
% f flags: immediate switch on first suspicion
if locked1 && locked2
    selected_sensor    = clamp(estimated_value, MIN_VAL, MAX_VAL);
    selected_sensor_id = 0;
    fault_flag         = 1;

elseif locked1 && ~locked2
    selected_sensor    = clamp(mn2, MIN_VAL, MAX_VAL);
    selected_sensor_id = 2;
    fault_flag         = 1;

elseif ~locked1 && locked2
    selected_sensor    = clamp(mn1, MIN_VAL, MAX_VAL);
    selected_sensor_id = 1;
    fault_flag         = 1;

else
    % Neither locked yet — switch immediately on suspicion
    if f1 && ~f2
        selected_sensor    = clamp(mn2, MIN_VAL, MAX_VAL);
        selected_sensor_id = 2;
        fault_flag         = 1;
    elseif f2 && ~f1
        selected_sensor    = clamp(mn1, MIN_VAL, MAX_VAL);
        selected_sensor_id = 1;
        fault_flag         = 1;
    elseif f1 && f2
        selected_sensor    = clamp(estimated_value, MIN_VAL, MAX_VAL);
        selected_sensor_id = 0;
        fault_flag         = 1;
    else
        selected_sensor    = clamp(mn1, MIN_VAL, MAX_VAL);
        selected_sensor_id = 1;
        fault_flag         = 0;
    end
end

end


function y = clamp(x, lo, hi)
    if x < lo;      y = lo;
    elseif x > hi;  y = hi;
    else;           y = x;
    end
end

== matlab function Full_Integration_Redundant/SbW Subsystem/Sensor_primary/MATLAB Function2 ==
  settings: updateMethod=DISCRETE
  data: sensor_in input; sensor_out output; fault_type input


function sensor_out = sensor_fault(sensor_in, fault_type)
% SENSOR_FAULT - Inject sensor faults via Step block
%
% Fault Types:
%   0 = Normal        - clean pass-through
%   1 = Bias          - constant offset added
%   2 = Noise         - random noise added
%   3 = Short Circuit - output forced to zero
%   4 = Drift         - gradual ramp added over time
%
% Connect a Step block to fault_type input:
%   Initial value = 0, Final value = 1/2/3/4

persistent drift_accumulator fault_active stuck_value

% INITIALISATION

if isempty(drift_accumulator)
    drift_accumulator = 0;
    fault_active      = false;
    stuck_value       = 0;
end

% PARAMETERS  – tune these to your signal range
BIAS_VALUE  = 5.0;    % Constant offset for bias fault
NOISE_STD   = 3.0;    % Standard deviation of injected noise
DRIFT_RATE  = 0.05;   % Drift added per sample when fault is active

% Box-Muller noise (replaces randn - works in Simulink Function blocks)
u1 = rand();
u2 = rand();
if u1 < 1e-10; u1 = 1e-10; end
noise = NOISE_STD * sqrt(-2.0 * log(u1)) * cos(2.0 * pi * u2);

% FAULT INJECTION
switch round(fault_type)

    case 0
        % NORMAL - clean signal, reset all fault states
        sensor_out        = sensor_in;
        drift_accumulator = 0;
        fault_active      = false;
        stuck_value       = 0;

    case 1
        % BIAS - fixed constant offset
        sensor_out = sensor_in + BIAS_VALUE;

    case 2
        % NOISE - random noise on every sample
        sensor_out = sensor_in + noise;

    case 3
        % SHORT CIRCUIT - output collapses to zero
        sensor_out = 0;

    case 4
        % DRIFT - ramp that grows from the moment Step fires
        if ~fault_active
            fault_active      = true;
            drift_accumulator = 0;   % start ramp from zero at fault onset
        end
        drift_accumulator = drift_accumulator + DRIFT_RATE;
        sensor_out        = sensor_in + drift_accumulator;

    otherwise
        sensor_out = sensor_in;

end
end
